simulink model "simple_relaxed_ANSFT"  (R2023a)
settings: Solver=ode4  StartTime=0.0  StopTime=72  FixedStep=0.01  RelTol=1e-3
model workspace (MAT data in the model file):
  tra1 = [0 2 0 -2 0 2]
  tra2 = [0 2 2 2 2 0]
  tra3 = [0 0 2 2 2 2]
  wn = 10
values from neighbouring files (symbols this model uses):
  F = 5    [assignment3.m]
undefined symbols (not defined in the file or in its folder): Light, MIL
libraries: dspsrcs4 x7, simulink x5, robotcorelib x1, aerolibwind2 x1
settings Model: Creator=Adan Daniel  LastModifiedBy=adan
settings OptimizationCC: ReuseModelBlockBuffer=off

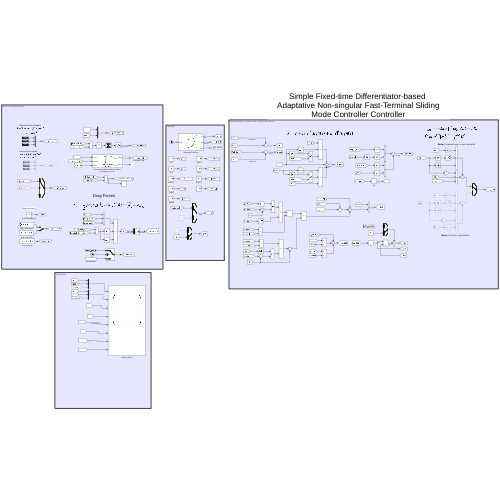
[thumbnail: Simulink's stored preview of the top-level diagram]
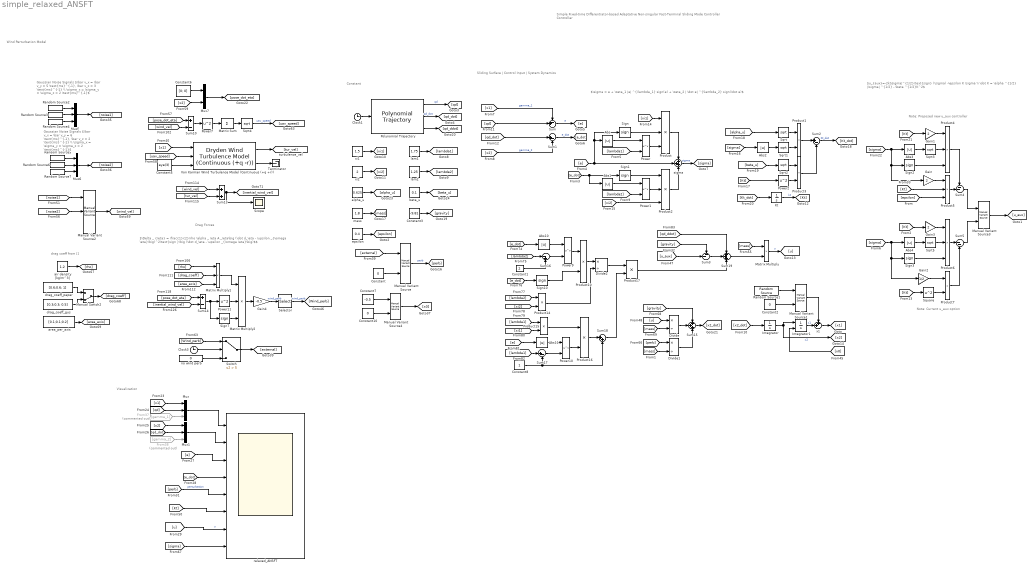
== system simple_relaxed_ANSFT ==
  note: Note: Current u_aux option
  note: Note: Proposed new u_aux controller
  note: Sliding Surface | Control Input | System Dynamics
  note: Constant
  note: Visualization
  note: Simple Fixed-time Differentiator-based
      | Adaptative Non-singular Fast-Terminal Sliding Mode Controller Controller
  note: $\sigma = e + \zeta_1 |e| ^{\lambda_1} sign(e) + \zeta_2 | \dot e| ^{\lambda_2} sign(\dot e)$
  note: $u_{aux}=-2k|\sigma|^{1/2}\text{sign} (\sigma) -\epsilon K \sigma \\ \dot K = \alpha ^{1/2} |\sigma| ^{1/2} - \beta ^{1/2}K^2$
  note: Gaussian Noise Signals
      | $\bar v_x = \bar v_y = 5 \text{ms}^{-1}, \bar v_z = 3 \text{ms}^{-1} \\ \sigma_x = \sigma_y = \sigma_z = 2 \text{ms}^{-1}$
  note: $\Delta _ {\eta} = \frac{1}{2}\rho \alpha _ \eta A _\eta\big (\dot d_\eta - \upsilon _{\omega \eta}\big)^2\text{sign }\big (\dot d_\eta - \upsilon _{\omega \eta}\big)$$
  note: drag coeff from []
  note: Gaussian Noise Signals
      | $\bar v_x = \bar v_y = 6 \text{ms}^{-1}, \bar v_z = 2 \text{ms}^{-1} \\ \sigma_x = \sigma_y = \sigma_z = 2 \text{ms}^{-1}$
  note: Wind Perturbation Model
  note: Drag Forces
  Abs{,1..4,10..11} (7 alike) : Abs  SaturateOnIntegerOverflow=off
  Clock1 : Clock
  Clock3 : Clock
  Constant : Constant  Value=0
  Constant1 : Constant  Value=2
  Constant10 : Constant  Value=0
  Constant2 : Constant  Value=0
  Constant3 : Constant  Value=-9.81
  Constant5 : Constant  Value=eye(3)
  Constant6 : Constant  Value=[0; 0]
  Constant7 : Constant  Value=-0.5
  Constant8 : Constant
  Divide : Product  Inputs=*/
  Divide1 : Product  Inputs=*/
  Divide2 : Product  Inputs=*/
  From37 : From  Commented=on  GotoTag=gamma_1
  From38 : From  Commented=on  GotoTag=gamma_2
  Gain : Gain  Gain=2
  Gain1 : Gain  Gain=2
  Gain2 : Gain  Gain=1/2
  Gain3 : Gain  Gain=2
  Gain4 : Gain  Gain=-0.5
  Integrator : Integrator
  Integrator1 : Integrator  InitialConditionSource=external
  Kt : Integrator
  Manual Variant Source : simulink/Signal Routing/Manual Variant Source  NumChoices=2  LabelModeActiveChoice=V_1
  Manual Variant Source1 : simulink/Signal Routing/Manual Variant Source  NumChoices=2  LabelModeActiveChoice=V_2
  Manual Variant Source2 : simulink/Signal Routing/Manual Variant Source  NumChoices=3  LabelModeActiveChoice=V_1
  Manual Variant Source3 : simulink/Signal Routing/Manual Variant Source  NumChoices=2  LabelModeActiveChoice=V_1
  Manual Variant Source4 : simulink/Signal Routing/Manual Variant Source  NumChoices=2  LabelModeActiveChoice=V_2
  Manual Switch2 : ManualSwitch  CurrentSetting=0
  Matrix Sum : Sum  Inputs=+
  Matrix Multiply : Product
  Matrix Multiply1 : Product  Inputs=3
  Matrix Multiply2 : Product  Inputs=3
  Mux{,1,5..6} (4 alike) : Mux  Inputs=3
  Mux7 : Mux  Inputs=2
  Polynomial Trajectory : robotcorelib/Polynomial Trajectory  WaypointSource=Internal  Waypoints=tra2  TimePoints=[0, 12, 24, 36, 48, 60]  TimeInterval=[ 1, 4 ]  Method=Cubic Polynomial  ParameterSource=Internal  VelocityBoundaryCondition=zeros( 1, 6 )  AccelerationBoundaryCondition=zeros( 2, 5 )  SimulateUsing=Interpreted execution
  Power{,1,9..10} (4 alike) : Math  Operator=pow
  Power11 : Math  Operator=square
  Power2 : Math  Operator=square
  Power7 : Math  Operator=square
  Product{,2,4..6} (5 alike) : Product  Inputs=3
  Product{1,3,7,10,14..17} (8 alike) : Product
  Random Source1 : dspsrcs4/Random Source  SrcType=Gaussian  NormMethod=Ziggurat  CltLength=12  MinVal=0  MaxVal=1  MeanVal=0.005  VarVal=0.001 * 0.001  RepMode=Not repeatable  rawSeed=1  IsInherit=off  SampMode=Continuous  SampTime=0.01  SampFrame=1  DataType=Double  OutComplex=Real  OutputFrames=off
  Random Source2 : dspsrcs4/Random Source  SrcType=Gaussian  NormMethod=Ziggurat  CltLength=12  MinVal=0  MaxVal=1  MeanVal=5  VarVal=2  RepMode=Not repeatable  rawSeed=1  IsInherit=off  SampMode=Discrete  SampTime=1  SampFrame=1  DataType=Double  OutComplex=Real  OutputFrames=off
  Random Source3 : dspsrcs4/Random Source  SrcType=Gaussian  NormMethod=Ziggurat  CltLength=12  MinVal=0  MaxVal=1  MeanVal=5  VarVal=2  RepMode=Not repeatable  rawSeed=1  IsInherit=off  SampMode=Discrete  SampTime=1  SampFrame=1  DataType=Double  OutComplex=Real  OutputFrames=off
  Random Source4 : dspsrcs4/Random Source  SrcType=Gaussian  NormMethod=Ziggurat  CltLength=12  MinVal=0  MaxVal=1  MeanVal=3  VarVal=2  RepMode=Specify seed  rawSeed=1  IsInherit=off  SampMode=Discrete  SampTime=1  SampFrame=1  DataType=Double  OutComplex=Real  OutputFrames=off
  Random Source5 : dspsrcs4/Random Source  SrcType=Gaussian  NormMethod=Ziggurat  CltLength=12  MinVal=0  MaxVal=1  MeanVal=6  VarVal=2  RepMode=Not repeatable  rawSeed=1  IsInherit=off  SampMode=Discrete  SampTime=1  SampFrame=1  DataType=Double  OutComplex=Real  OutputFrames=off
  Random Source6 : dspsrcs4/Random Source  SrcType=Gaussian  NormMethod=Ziggurat  CltLength=12  MinVal=0  MaxVal=1  MeanVal=6  VarVal=2  RepMode=Not repeatable  rawSeed=1  IsInherit=off  SampMode=Discrete  SampTime=1  SampFrame=1  DataType=Double  OutComplex=Real  OutputFrames=off
  Random Source7 : dspsrcs4/Random Source  SrcType=Gaussian  NormMethod=Ziggurat  CltLength=12  MinVal=0  MaxVal=1  MeanVal=2  VarVal=2  RepMode=Not repeatable  rawSeed=1  IsInherit=off  SampMode=Discrete  SampTime=1  SampFrame=1  DataType=Double  OutComplex=Real  OutputFrames=off
  Scope : Scope
  Selector : Selector  InputPortWidth=3  IndexOptions=Index vector (dialog)  Indices=[3]  OutputSizes=1
  Sign{,1..3,7,10} (6 alike) : Signum
  Sqrt{,1..5} (6 alike) : Sqrt
  Square : Math  Operator=square
  Sum : Sum  Inputs=-+|
  Sum1 : Sum  Inputs=|+-
  Sum10 : Sum  Inputs=+-
  Sum13 : Sum
  Sum14 : Sum  Inputs=+-
  Sum15 : Sum  Inputs=+++
  Sum16 : Sum  Inputs=|-+
  Sum17 : Sum  Inputs=|+-
  Sum18 : Sum  Inputs=|++
  Sum19 : Sum  Inputs=+++
  Sum2 : Sum  Inputs=|+-
  Sum3 : Sum  Inputs=--|
  Sum4 : Sum  Inputs=--|
  Sum5 : Sum  Inputs=|--
  Switch : Switch  Criteria=u2 > Threshold  Threshold=5  SaturateOnIntegerOverflow=off  InputSameDT=off
  Terminator : Terminator
  Von Karman Wind Turbulence Model (Continuous (+q +r)) : aerolibwind2/Dryden Wind Turbulence Model  (Continuous (+q -r))  units=Metric (MKS)  spec=MIL-F-8785C  model=Continuous Von Karman (+q +r)  W20=15  Wdeg=0  TurbProb=10^-2 - Light  L_high=762  Wingspan=10  ts=0.1  Seed=[23341 23342 23343 23344]  T_on=on
      settings: LibrarySourceBlock=|
      | aerolibwind2/Von Karman Wind Turbulence Model
      | (Continuous (+q +r))
  air density [kg/m^3] : Constant  Value=1.2
  alpha_u : Constant  Value=0.625
  area_per_axis : Constant  Value=[0.1;0.1;0.2]
  beta_u : Constant  Value=0.1
  drag_coeff_gus : Constant  Value=[0.3;0.3; 0.5]
  drag_coeff_paper : Constant  Value=[0.6;0.6; 1]
  epsilon : Constant  Value=0.4
  lam1 : Constant  Value=1.75
  lam2 : Constant  Value=1.25
  mass : Constant  Value=1.8
  no wind perb : Constant  Value=0
  relaxed_ANSFT : Scope  NumInputPorts=8
  sigma : Sum  Inputs=+++
  x1 : Sum  Inputs=++|
  xi1 : Constant  Value=1.5
  xi2 : Constant  Value=2
  wires:
  Integrator/1 -> [x2], Integrator1/1  "x2"
  Sum1/1 -> [e_dot]  "e_dot"
  Mux/1 -> relaxed_ANSFT/1
  [x2_dot] -> Integrator/1
  Clock1/1 -> Polynomial Trajectory/1
  Polynomial Trajectory/3 -> [qd_ddot]
  [qd] -> Mux/2
  Polynomial Trajectory/1 -> [qd]  "qd"
  Polynomial Trajectory/2 -> [qd_dot]  "qd_dot"
  [qd] -> Sum/2
  [qd_dot] -> Sum1/1
  Sum/1 -> [e]  "e"
  lam1/1 -> [lambda1]
  lam2/1 -> [lambda2]
  xi1/1 -> [xi1]
  xi2/1 -> [xi2]
  [x1] -> Mux/1
  [qd_dot] -> Mux1/2
  [x2] -> Mux1/1
  Mux1/1 -> relaxed_ANSFT/2
  [e] -> relaxed_ANSFT/3
  [e_dot] -> relaxed_ANSFT/4
  [perb] -> relaxed_ANSFT/5  "perturbation"
  Manual Variant Source/1 -> [perb]  "perb"
  mass/1 -> [mass]
  From37/1 -> Mux/3
  From38/1 -> Mux1/3
  [x1] -> Sum/1  "gamma_1"
  [x2] -> Sum1/2  "gamma_2"
  Constant3/1 -> [gravity]
  [u] -> Divide/1
  [e] -> sigma/2, Abs/1, Sign/1
  Abs/1 -> Power/1
  [lambda1] -> Power/2
  Power/1 -> Product/3
  Sign/1 -> Product/2
  sigma/1 -> [sigma]  "sigma"
  Power1/1 -> Product2/2
  [e_dot] -> Abs1/1, Sign1/1
  [lambda2] -> Power1/2
  Abs1/1 -> Power1/1
  Sign1/1 -> Product2/1
  Product2/1 -> sigma/3
  Product/1 -> sigma/1
  [xi1] -> Product/1
  [xi2] -> Product2/3
  beta_u/1 -> [beta_u]
  alpha_u/1 -> [alpha_u]
  [Kt] -> Power2/1
  [alpha_u] -> Sqrt/1
  [sigma] -> Abs2/1
  Abs2/1 -> Sqrt1/1
  Sqrt1/1 -> Product1/2
  Power2/1 -> Product3/2
  [beta_u] -> Sqrt2/1
  Sqrt/1 -> Product1/1
  Product3/1 -> Sum2/2
  Product1/1 -> Sum2/1
  Sqrt2/1 -> Product3/1
  Sum2/1 -> [Kt_dot]  "Kt_dot"
  [Kt_dot] -> Kt/1
  Kt/1 -> [Kt]  "kt"
  Sqrt3/1 -> Product4/2
  Product4/1 -> Sum4/1
  Abs3/1 -> Sqrt3/1
  [Kt] -> Gain1/1
  Sign2/1 -> Product4/3
  [Kt] -> Product5/2
  [sigma] -> Abs3/1, Gain/1, Sign2/1
  Product5/1 -> Sum4/2
  Sum4/1 -> Manual Variant Source3/1
  Matrix Multiply/1 -> [u]  "u"
  Sum15/1 -> [x2_dot]
  [mass] -> Divide/2
  Divide/1 -> Sum15/2
  [perb] -> Divide1/1
  [gravity] -> Sum15/1
  [mass] -> Matrix Multiply/1
  [u_aux] -> Sum3/2
  [e_dot] -> Abs10/1
  Sum16/1 -> Power9/2
  Sign10/1 -> Product10/2
  Abs10/1 -> Power9/1
  Product14/1 -> Divide2/2
  Constant1/1 -> Sum16/2
  [lambda2] -> Sum16/1
  Power9/1 -> Product10/1
  [lambda2] -> Product14/1
  [e_dot] -> Sign10/1
  Product10/1 -> Divide2/1
  [xi2] -> Product14/2
  Product15/1 -> Product16/1
  Product16/1 -> Sum18/1
  Power10/1 -> Product16/2
  Constant8/1 -> Sum18/2, Sum17/2
  [xi1] -> Product15/2
  [lambda1] -> Product15/1
  Abs11/1 -> Power10/1
  [lambda1] -> Sum17/1
  [e] -> Abs11/1
  Sum17/1 -> Power10/2
  Divide2/1 -> Product17/1
  Sum18/1 -> Product17/2
  Sum19/1 -> Matrix Multiply/2
  Sum3/1 -> Sum19/2
  Product17/1 -> Sum19/3
  [qd_ddot] -> Sum19/1
  [gravity] -> Sum3/1
  Constant2/1 -> Manual Variant Source1/2
  Random Source1/1 -> Manual Variant Source1/1
  Integrator1/1 -> x1/2  "x1"
  x1/1 -> [x1]
  Manual Variant Source1/1 -> x1/1
  drag_coeff_gus/1 -> Manual Switch2/2
  [uav_speed] -> Von Karman Wind Turbulence Model (Continuous (+q +r))/2
  [x2] -> Mux7/2
  Random Source2/1 -> Mux5/1
  Constant6/1 -> Mux7/1
  Sqrt4/1 -> [uav_speed]  "uav_speed"
  [noise1] -> Manual Variant Source2/1
  Random Source3/1 -> Mux5/2
  Random Source5/1 -> Mux6/1
  area_per_axis/1 -> [area_axis]
  [x1] -> Von Karman Wind Turbulence Model (Continuous (+q +r))/1
  [area_axis] -> Matrix Multiply1/3
  [inertial_wind_vel] -> Sum14/2
  Sign7/1 -> Matrix Multiply2/3
  no wind perb/1 -> Switch/3
  [wind_vel] -> Sum13/1
  Matrix Multiply2/1 -> Gain4/1
  [drag_coeff] -> Matrix Multiply1/2
  Gain4/1 -> Selector/1  "wind_perb"
  Manual Switch2/1 -> [drag_coeff]
  [tur_vel] -> Sum13/2
  Manual Variant Source2/1 -> [wind_vel]
  [rho] -> Matrix Multiply1/1
  Selector/1 -> [Wind_perb]  "wind_perb"
  Matrix Multiply1/1 -> Matrix Multiply2/1
  Sum10/1 -> Power7/1
  Power11/1 -> Matrix Multiply2/2
  Clock3/1 -> Switch/2
  Switch/1 -> [external]
  Mux5/1 -> [noise1]
  Sum14/1 -> Sign7/1, Power11/1
  Von Karman Wind Turbulence Model (Continuous (+q +r))/1 -> [tur_vel]
  [noise2] -> Manual Variant Source2/2
  Constant5/1 -> Von Karman Wind Turbulence Model (Continuous (+q +r))/3
  Mux7/1 -> [pose_dot_eta]
  [Wind_perb] -> Switch/1
  Random Source4/1 -> Mux5/3
  [pose_dot_eta] -> Sum14/1
  Power7/1 -> Matrix Sum/1
  air density [kg/m^3]/1 -> [rho]
  Matrix Sum/1 -> Sqrt4/1
  drag_coeff_paper/1 -> Manual Switch2/1
  Random Source6/1 -> Mux6/2
  Sum13/1 -> Scope/1, [inertial_wind_vel]
  Random Source7/1 -> Mux6/3
  Mux6/1 -> [noise2]
  [pose_dot_eta] -> Sum10/1
  [wind_vel] -> Sum10/2
  Von Karman Wind Turbulence Model (Continuous (+q +r))/2 -> Terminator/1
  Constant10/1 -> Manual Variant Source4/2
  Manual Variant Source4/1 -> [x0]
  Constant7/1 -> Manual Variant Source4/1
  [x0] -> Integrator1/2
  epsilon/1 -> [epsilon]
  [epsilon] -> Product5/3
  Gain/1 -> Product5/1
  Gain1/1 -> Product4/1
  [u] -> relaxed_ANSFT/7  "u"
  [sigma] -> relaxed_ANSFT/8
  [Kt] -> relaxed_ANSFT/6
  Sqrt5/1 -> Product6/2
  [Kt] -> Square/1
  [Kt] -> Gain3/1
  Sign3/1 -> Product6/3
  Abs4/1 -> Sqrt5/1
  Gain3/1 -> Product6/1
  Gain2/1 -> Product7/1
  Product6/1 -> Sum5/1
  Product7/1 -> Sum5/2
  [sigma] -> Abs4/1, Gain2/1, Sign3/1
  Sum5/1 -> Manual Variant Source3/2
  Manual Variant Source3/1 -> [u_aux]
  Square/1 -> Product7/2
  [mass] -> Divide1/2
  Divide1/1 -> Sum15/3
  [external] -> Manual Variant Source/1
  Constant/1 -> Manual Variant Source/2
